simulink model "SigNetLabExp3code_19CS10044"  (R2020b)
settings: Solver=ode23t  StartTime=0.0  StopTime=10.0  RelTol=1e-3
libraries: powerlib x9, powerlib_meascontrol x2
settings Model: Creator=mluser  LastModifiedBy=mluser

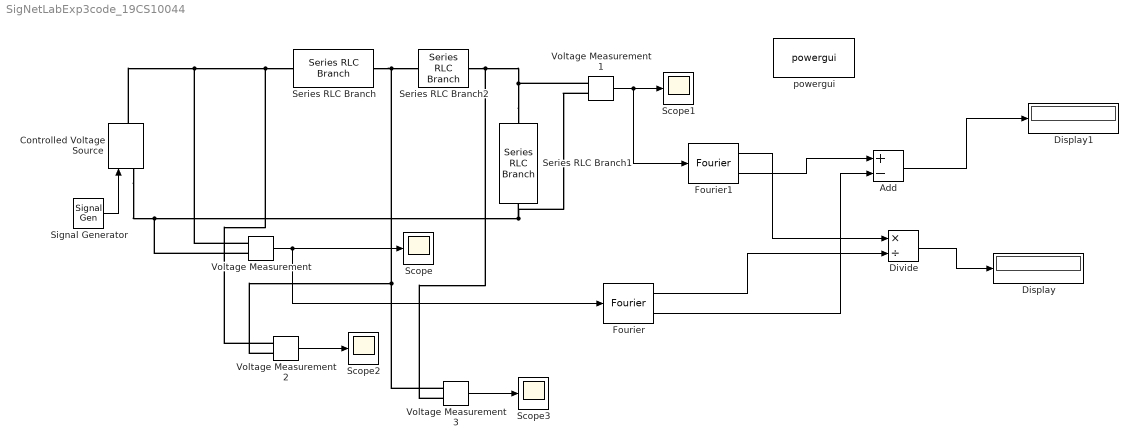
== system SigNetLabExp3code_19CS10044 ==
  Add : Sum  Inputs=+-
  Controlled Voltage Source : powerlib/Electrical Sources/Controlled Voltage Source  Initialize=on  Source_Type=AC  Amplitude=1  Phase=0  Frequency=100  Measurements=None
  Display : Display
  Display1 : Display
  Divide : Product  Inputs=*/
  Fourier : powerlib_meascontrol/Measurements/Fourier  Freq=100  n=1  InInit=[0, 0]  Ts=0
  Fourier1 : powerlib_meascontrol/Measurements/Fourier  Freq=100  n=1  InInit=[0, 0]  Ts=0
  Scope{,1..3} (4 alike) : Scope
  Series RLC Branch : powerlib/Elements/Series RLC Branch  LConnTagsString=__new0  RConnTagsString=__new0  BranchType=R  Resistance=400  Inductance=0.1  SetiL0=off  InitialCurrent=0  Capacitance=1e-6  Setx0=off  InitialVoltage=0  Measurements=None
  Series RLC Branch1 : powerlib/Elements/Series RLC Branch  LConnTagsString=__new0  RConnTagsString=__new0  BranchType=C  Resistance=1  Inductance=1e-3  SetiL0=off  InitialCurrent=0  Capacitance=1e-7  Setx0=off  InitialVoltage=0  Measurements=None
  Series RLC Branch2 : powerlib/Elements/Series RLC Branch  LConnTagsString=__new0  RConnTagsString=__new0  BranchType=L  Resistance=1  Inductance=0.1  SetiL0=off  InitialCurrent=0  Capacitance=1e-6  Setx0=off  InitialVoltage=0  Measurements=None
  Signal Generator : SignalGenerator  Frequency=100
  Voltage Measurement{,1..3} (4 alike) : powerlib/Measurements/Voltage Measurement  PhasorSimulation=off  OutputType=Complex  PSBequivalent=0
  powergui : powerlib/powergui  Priority=1  SimulationMode=Continuous  SampleTime=50e-6  frequency=60  Iterations=50  frequencyindice=100  Pbase=100e6  ErrMax=1e-4  UnitsV=kV  UnitsW=MW  buscounter=0  FunctionMessages=off  echomessages=off  EnableUseOfTLC=off  CurrentSourceSwitches=off  DisableSnubberDevices=off  DisableRonSwitches=off  DisableVfSwitches=off  DisplayEquations=off  AutomaticDiscreteSolvers=off  SolverType=Tustin/Backward Euler (TBE)  Interpol=off  ExternalGateDelay=off  methode=off  Ts=100  x0status=blocks  SPID=on  SwTol=0  HookPort=off  NonlinearTolerance=1e-4  nMaxIteration=100  ContinueOnMaxIteration=off  RestoreLinks=warning  ResistiveCurrentMeasurement=off  Frange=[0:2:500]  Ylog=off  Xlog=on  ShowGrid=off  save=off  variable=ZData  structure=0  ZoomFFT=off  StartTime=0.0  cycles=1  DisplayStyle=1  fundamental=60  FreqAxis=off  MaxFrequency=1000  frequencyindicesteady=1  RmsSteady=1  display=off
  wires:
  Signal Generator/1 -> Controlled Voltage Source/1
  Voltage Measurement/1 -> Scope/1, Fourier/1
  Voltage Measurement1/1 -> Fourier1/1, Scope1/1
  Fourier1/2 -> Add/1
  Fourier/2 -> Add/2
  Fourier1/1 -> Divide/1
  Fourier/1 -> Divide/2
  Add/1 -> Display1/1
  Divide/1 -> Display/1
  Voltage Measurement2/1 -> Scope2/1
  Voltage Measurement3/1 -> Scope3/1
  connections:
  Controlled Voltage Source/RConn1 -- Voltage Measurement/LConn1 -- Voltage Measurement2/LConn1 -- Series RLC Branch/LConn1
  Series RLC Branch1/LConn1 -- Voltage Measurement3/LConn2 -- Series RLC Branch2/RConn1 -- Voltage Measurement1/LConn1
  Controlled Voltage Source/LConn1 -- Voltage Measurement/LConn2 -- Voltage Measurement1/LConn2 -- Series RLC Branch1/RConn1
  Series RLC Branch/RConn1 -- Voltage Measurement2/LConn2 -- Voltage Measurement3/LConn1 -- Series RLC Branch2/LConn1
